simulink model "SimProceso"  (R2023b)
settings: Solver=VariableStepAuto  StartTime=0.0  StopTime=1080  RelTol=1e-3
libraries: simulink x2
settings Model: Creator=alexa  LastModifiedBy=alexa

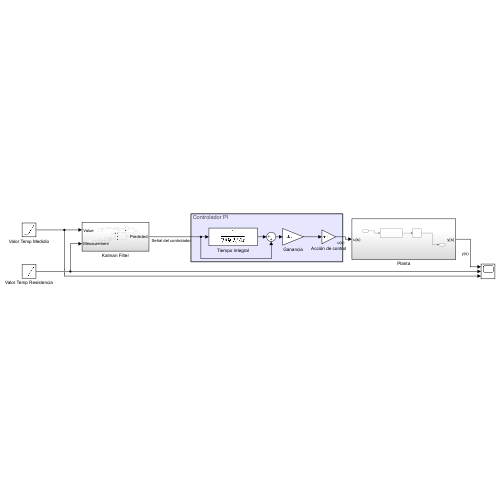
[thumbnail: Simulink's stored preview of the top-level diagram]
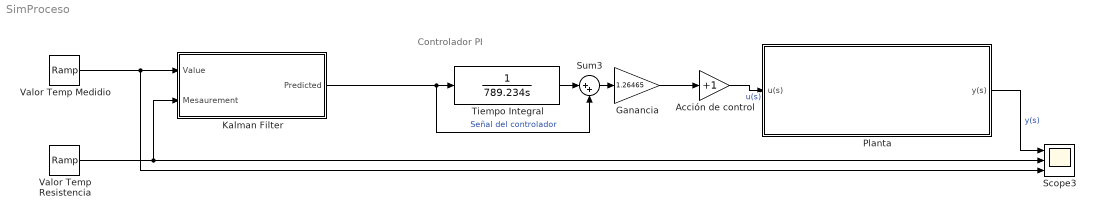
== system SimProceso ==
  note: Controlador PI
  Acción de control : Gain  Gain=+1
  Ganancia : Gain  Gain=1.26465
  Kalman Filter : Subsystem
  Planta : Subsystem
  Scope3 : Scope  NumInputPorts=3
  Sum3 : Sum  Inputs=|++
  Tiempo Integral : TransferFcn  Denominator=[789.234 0]
  Valor Temp Medidio : simulink/Sources/Ramp  slope=0.05  start=100  InitialOutput=20
  Valor Temp Resistencia : simulink/Sources/Ramp  slope=0.05  start=40  InitialOutput=20
  wires:
  Kalman Filter/1(Predicted) -> Sum3/2, Tiempo Integral/1  "Señal del controlador"
  Valor Temp Resistencia/1 -> Scope3/2, Kalman Filter/2(Mesaurement)
  Valor Temp Medidio/1 -> Kalman Filter/1(Value), Scope3/3
  Tiempo Integral/1 -> Sum3/1
  Sum3/1 -> Ganancia/1
  Ganancia/1 -> Acción de control/1
  Acción de control/1 -> Planta/1(u(s))  "u(s)"
  Planta/1(y(s)) -> Scope3/1  "y(s)"

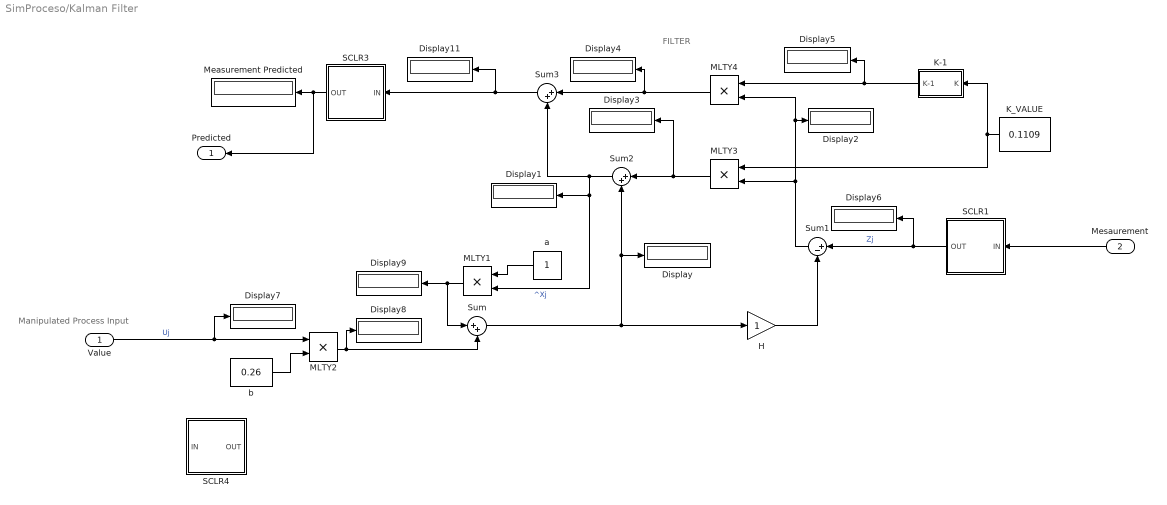
== system SimProceso/Kalman Filter ==
  note: FILTER
  note: Manipulated
      | Process
      | Input
  Value : Inport
  Mesaurement : Inport  Port=2
  " Measurement Predicted" : Display
  Display{,1..9,11} (11 alike) : Display
  H : Gain
  K-1 : Subsystem
  K_VALUE : Constant  Value=0.1109
  MLTY{1..4} (4 alike) : Product
  SCLR1 : Subsystem
  SCLR3 : Subsystem
  SCLR4 : Subsystem
  Sum : Sum  Inputs=|++
  Sum1 : Sum  Inputs=|+-
  Sum2 : Sum  Inputs=|++
  Sum3 : Sum  Inputs=|++
  a : Constant
  b : Constant  Value=0.26
  Predicted : Outport
  wires:
  Value/1 -> MLTY2/1, Display7/1  "Uj"
  Sum1/1 -> Display2/1, MLTY4/2, MLTY3/2
  H/1 -> Sum1/2
  MLTY4/1 -> Display4/1, Sum3/1
  MLTY2/1 -> Sum/2, Display8/1
  a/1 -> MLTY1/1
  Sum/1 -> H/1, Display/1, Sum2/2
  MLTY1/1 -> Sum/1, Display9/1
  SCLR1/1(OUT) -> Sum1/1, Display6/1  "Zj"
  Sum2/1 -> MLTY1/2, Display1/1, Sum3/2  "^Xj"
  SCLR3/1(OUT) -> Predicted/1, " Measurement Predicted"/1
  K-1/1(K-1) -> Display5/1, MLTY4/1
  MLTY3/1 -> Sum2/1, Display3/1
  Sum3/1 -> Display11/1, SCLR3/1(IN)
  K_VALUE/1 -> K-1/1(K), MLTY3/1
  b/1 -> MLTY2/2
  Mesaurement/1 -> SCLR1/1(IN)

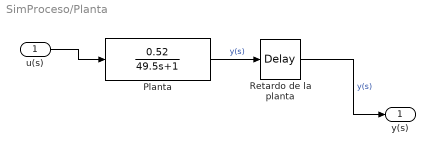
== system SimProceso/Planta ==
  u(s) : Inport
  Planta : TransferFcn  Numerator=[0.52]  Denominator=[49.5 1]
  Retardo de la planta : TransportDelay  DelayTime=129
  y(s) : Outport
  wires:
  Planta/1 -> Retardo de la planta/1  "y(s)"
  u(s)/1 -> Planta/1
  Retardo de la planta/1 -> y(s)/1  "y(s)"

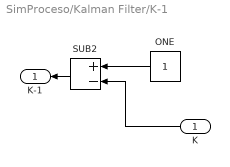
== system SimProceso/Kalman Filter/K-1 ==
  K : Inport
  ONE : Constant
  SUB2 : Sum  Inputs=+-
  K-1 : Outport
  wires:
  SUB2/1 -> K-1/1
  ONE/1 -> SUB2/1
  K/1 -> SUB2/2

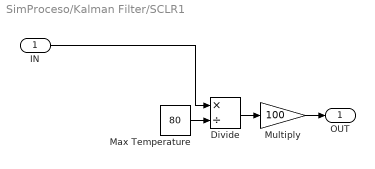
== system SimProceso/Kalman Filter/SCLR1 ==
  IN : Inport
  Divide : Product  Inputs=*/
  Max Temperature : Constant  Value=80
  Multiply : Gain  Gain=100
  OUT : Outport
  wires:
  Max Temperature/1 -> Divide/2
  Divide/1 -> Multiply/1
  IN/1 -> Divide/1
  Multiply/1 -> OUT/1

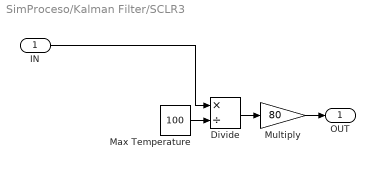
== system SimProceso/Kalman Filter/SCLR3 ==
  IN : Inport
  Divide : Product  Inputs=*/
  Max Temperature : Constant  Value=100
  Multiply : Gain  Gain=80
  OUT : Outport
  wires:
  Max Temperature/1 -> Divide/2
  Divide/1 -> Multiply/1
  IN/1 -> Divide/1
  Multiply/1 -> OUT/1

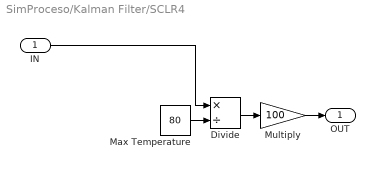
== system SimProceso/Kalman Filter/SCLR4 ==
  IN : Inport
  Divide : Product  Inputs=*/
  Max Temperature : Constant  Value=80
  Multiply : Gain  Gain=100
  OUT : Outport
  wires:
  Max Temperature/1 -> Divide/2
  Divide/1 -> Multiply/1
  IN/1 -> Divide/1
  Multiply/1 -> OUT/1
